simulink model "Robotics_KalmanFilter_example"  (R2022b)
settings: Solver=ode45  StartTime=0.0  StopTime=30  MaxStep=0.01  RelTol=1e-3
libraries: dspmathops x1
settings Model: Creator=score  LastModifiedBy=zhouwenjie
settings OptimizationCC: ReuseModelBlockBuffer=on

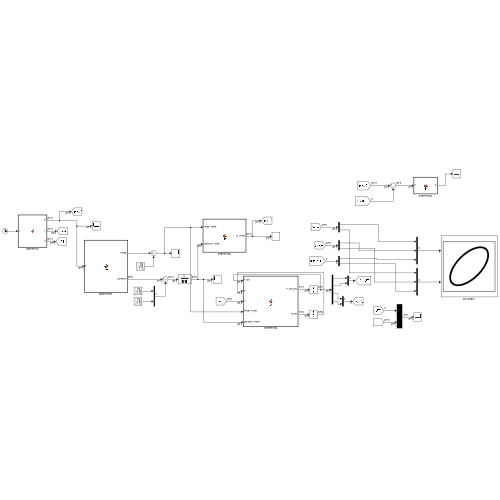
[thumbnail: Simulink's stored preview of the top-level diagram]
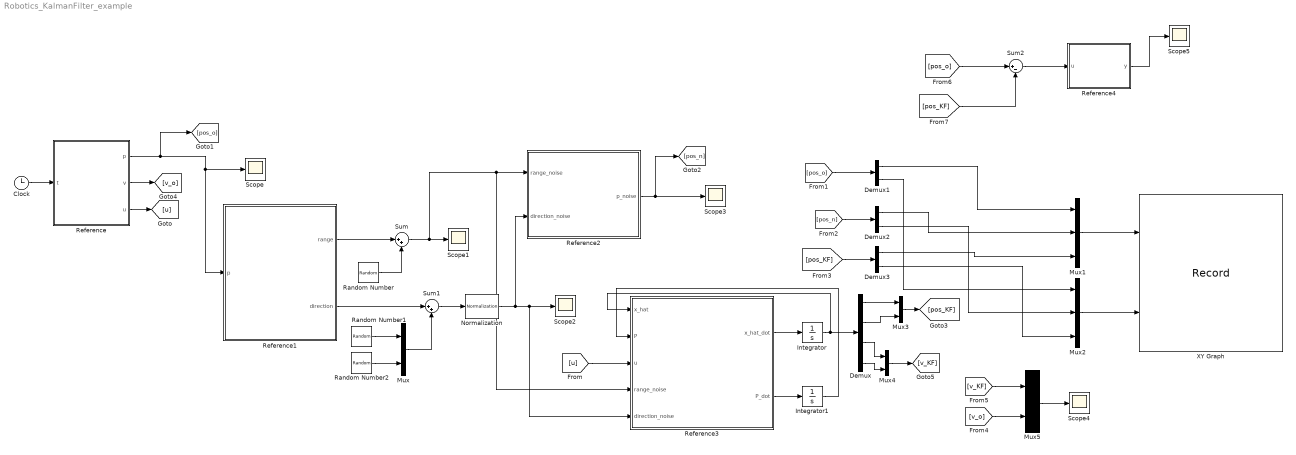
== system Robotics_KalmanFilter_example ==
  Clock : Clock
  Demux : Demux
  Demux1 : Demux  Outputs=2
  Demux2 : Demux  Outputs=2
  Demux3 : Demux  Outputs=2
  Integrator : Integrator  InitialCondition=[-3; -3; 0; 0]
  Integrator1 : Integrator  InitialCondition=100*eye(4)
  Mux{,3..5} (4 alike) : Mux  Inputs=2
  Mux1 : Mux  Inputs=3
  Mux2 : Mux  Inputs=3
  Normalization : dspmathops/Normalization  NormType=2-norm  Bias=1e-10  NormOver=Each column  Dimension=1  roundingMode=Floor  overflowMode=off  accumDataTypeStr=Inherit: Same as product output  accumLastDataTypeStr=Inherit: Same as product output  outputDataTypeStr=Inherit: Same as product output  outputMin=[]  outputMax=[]  outputLastDataTypeStr=Inherit: Same as product output
  Random Number : RandomNumber  Variance=0.01  Seed=randi(1000)  SampleTime=0.01
  Random Number1 : RandomNumber  Variance=0.01  Seed=randi(2000)  SampleTime=0.01
  Random Number2 : RandomNumber  Variance=0.01  Seed=randi(10000)  SampleTime=0.01
  Reference : MATLAB Function  TreatAsAtomicUnit=on
  Reference1 : MATLAB Function  TreatAsAtomicUnit=on
  Reference2 : MATLAB Function  TreatAsAtomicUnit=on
  Reference3 : MATLAB Function  TreatAsAtomicUnit=on
  Reference4 : MATLAB Function  TreatAsAtomicUnit=on
  Scope{,1..5} (6 alike) : Scope
  Sum : Sum  Inputs=|++
  Sum1 : Sum  Inputs=|++
  Sum2 : Sum  Inputs=|+-
  XY Graph : Record  FileSettingsInternal="{\"entries\":[{\"content\":{\"excelSettings\":{\"content\":{},\"type\":\"Streamout.ExcelSettings\"}},\"type\":\"Streamout.FileSettingStorage\",\"uuid\":\"99ddf482-bfd5-4986-8ef2-d08f1135ea4a\"}],\"packageUris\":[\"http://schema.mathworks.com/mf0/streamout_blocks/R2020a\"],\"version\":\"1.0\"}"  Layout=[1 1]  SignalsInternal="{\"entries\":[{\"content\":{\"signals\":[{\"content\":{\"blockPath\":[\"Robotics_KalmanFilter_example/XY Graph\"],\"channel\":[],\"dimensions\":[3],\"domain\":\"Robotics_KalmanFilter_example/XY Graph\",\"hasChildren\":true,\"lineColor\":\"#77ac30\",\"plots\":[],\"port\":1,\"sid\":[\"\"],\"signalID\":486,\"signalName\":\"Mux1\"},\"type\":\"RecordBlkView.Signal\",\"uuid\":\"85c66cea-82c2-4576-a2a4-b02d7115ceed\"},{\"content\":{\"blockPath\":[\"Robotics_KalmanFilter_example/XY Graph\"],\"channel\":[1],\"dimensions\":[3],\"domain\":\"Robotics_KalmanFilter_example/XY Graph\",\"lineColor\":\"#4dbeee\",\"parentID\":486,\"plots\":[1],\"port\":1,\"sid\":[\"\"],\"signalID\":487,\"signalName\":\"Mux1\"},\"type\":\"RecordBlkView.Signal\",\"uuid\":\"cc40eaf1-a560-40e5-9d45-80ed3782b7a2\"},{\"content\":{\"blockPath\":[\"Robotics_KalmanFilter_example/XY Graph\"],\"channel\":[],\"dimensions\":[3],\"domain\":\"Robotics_KalmanFilter_example/XY Graph\",\"hasChildren\":true,\"lineColor\":\"#a2142f\",\"plots\":[],\"port\":2,\"sid\":[\"\"],\"signalID\":491,\"signalName\":\"Mux2\"},\"type\":\"RecordBlkView.Signal\",\"uuid\":\"08abc5d3-c380-4d97-8386-a1200ecf61fc\"},{\"content\":{\"blockPath\":[\"Robotics_KalmanFilter_example/XY Graph\"],\"channel\":[1],\"dimensions\":[3],\"domain\":\"Robotics_KalmanFilter_example/XY Graph\",\"lineColor\":\"#139fff\",\"parentID\":491,\"plots\":[1],\"port\":2,\"sid\":[\"\"],\"signalID\":492,\"signalName\":\"Mux2\"},\"type\":\"RecordBlkView.Signal\",\"uuid\":\"281db55c-b3c3-4430-b4b5-2a782cee91c7\"},{\"content\":{\"blockPath\":[\"Robotics_KalmanFilter_example/XY Graph\"],\"channel\":[2],\"dimensions\":[3],\"domain\":\"Robotics_KalmanFilter_example/XY Graph\",\"lineColor\":\"#ff6929\",\"parentID\":486,\"plots\":[1],\"port\":1,\"sid\":[\"\"],\"signalID\":496,\"signalName\":\"Mux1\"},\"type\":\"RecordBlkView.Signal\",\"uuid\":\"7a39d2fa-2334-4a71-8704-de6660aef924\"},{\"content\":{\"blockPath\":[\"Robotics_KalmanFilter_example/XY Graph\"],\"channel\":[3],\"dimensions\":[3],\"domain\":\"Robotics_KalmanFilter_example/XY Graph\",\"lineColor\":\"#b746ff\",\"parentID\":486,\"plots\":[1],\"port\":1,\"sid\":[\"\"],\"signalID\":497,\"signalName\":\"Mux1\"},\"type\":\"RecordBlkView.Signal\",\"uuid\":\"9c037c13-9f68-4801-a7b2-66cb5fafd5da\"},{\"content\":{\"blockPath\":[\"Robotics_KalmanFilter_example/XY Graph\"],\"channel\":[2],\"dimensions\":[3],\"domain\":\"Robotics_KalmanFilter_example/XY Graph\",\"lineColor\":\"#64d413\",\"parentID\":491,\"plots\":[1],\"port\":2,\"sid\":[\"\"],\"signalID\":498,\"signalName\":\"Mux2\"},\"type\":\"RecordBlkView.Signal\",\"uuid\":\"d5859256-777d-4e96-97fc-4e17bee01a9a\"},{\"content\":{\"blockPath\":[\"Robotics_KalmanFilter_example/XY Graph\"],\"channel\":[3],\"dimensions\":[3],\"domain\":\"Robotics_KalmanFilter_example/XY Graph\",\"lineColor\":\"#ff13a6\",\"parentID\":491,\"plots\":[1],\"port\":2,\"sid\":[\"\"],\"signalID\":499,\"signalName\":\"Mux2\"},\"type\":\"RecordBlkView.Signal\",\"uuid\":\"d73878a8-5330-4d11-8cb2-697f64e39e63\"}]},\"type\":\"RecordBlkView.InputSignals\",\"uuid\":\"f320aaa5-5c90-4b2a-a994-0aa79a653834\"}],\"packageUris\":[\"http://schema.mathworks.com/mf0/streamout_blocks/R2020a\"],\"version\":\"1.0\"}"  VisualizationBindings="{\"xyplotplugin\":{\"info\":[{\"series\":[{\"bindingParametersList\":[{\"parameter\":\"X-Axis\",\"signalID\":496,\"signalName\":\"Mux1(2)\"},{\"parameter\":\"Y-Axis\",\"signalID\":498,\"signalName\":\"Mux2(2)\"}],\"seriesID\":37893},{\"bindingParametersList\":[{\"parameter\":\"X-Axis\",\"signalID\":487,\"signalName\":\"Mux1(1)\"},{\"parameter\":\"Y-Axis\",\"signalID\":492,\"signalName\":\"Mux2(1)\"}],\"seriesID\":24155},{\"bindingParametersList\":[{\"parameter\":\"X-Axis\",\"signalID\":497,\"signalName\":\"Mux1(3)\"},{\"parameter\":\"Y-Axis\",\"signalID\":499,\"signalName\":\"Mux2(3)\"}],\"seriesID\":670}],\"subplotID\":1}]}}"  CompatibilityTag=XY
  wires:
  Clock/1 -> Reference/1(t)
  Reference/1(p) -> [pos_o], Reference1/1(p), Scope/1
  Reference1/1(range) -> Sum/1
  Random Number/1 -> Sum/2
  Reference1/2(direction) -> Sum1/1
  Random Number1/1 -> Mux/1
  Random Number2/1 -> Mux/2
  Mux/1 -> Sum1/2
  Sum1/1 -> Normalization/1
  Sum/1 -> Reference2/1(range_noise), Reference3/4(range_noise), Scope1/1
  Normalization/1 -> Reference2/2(direction_noise), Reference3/5(direction_noise), Scope2/1
  Reference2/1(p_noise) -> [pos_n], Scope3/1
  Reference3/1(x_hat_dot) -> Integrator/1
  Reference3/2(P_dot) -> Integrator1/1
  Integrator1/1 -> Reference3/2(P)
  Integrator/1 -> Reference3/1(x_hat), Demux/1
  Reference/3(u) -> [u]
  [u] -> Reference3/3(u)
  Mux1/1 -> XY Graph/1
  Mux2/1 -> XY Graph/2
  Demux/1 -> Mux3/1
  Demux/2 -> Mux3/2
  Mux3/1 -> [pos_KF]
  [pos_o] -> Demux1/1
  [pos_n] -> Demux2/1
  [pos_KF] -> Demux3/1
  Demux1/1 -> Mux1/1
  Demux2/1 -> Mux1/2
  Demux3/1 -> Mux1/3
  Demux1/2 -> Mux2/1
  Demux2/2 -> Mux2/2
  Demux3/2 -> Mux2/3
  Reference/2(v) -> [v_o]
  Demux/3 -> Mux4/1
  Mux4/1 -> [v_KF]
  Demux/4 -> Mux4/2
  [v_KF] -> Mux5/1
  [v_o] -> Mux5/2
  Mux5/1 -> Scope4/1
  [pos_o] -> Sum2/1
  [pos_KF] -> Sum2/2
  Sum2/1 -> Reference4/1(u)
  Reference4/1(y) -> Scope5/1

== matlab function Robotics_KalmanFilter_example/Reference1 ==
  data: p input; range output; direction output
function [range, direction] = fcn(p)

range = norm(p);
direction = p/range;

== matlab function Robotics_KalmanFilter_example/Reference ==
  data: t input; p output; v output; u output
function [p, v, u] = fcn(t)

a = 1/2;
b = 1;
alpha = 1;
beta = -1/3;

p = [a*cos(alpha*t);
     b*sin(beta*t)];

v = [-a*alpha*sin(alpha*t);
     b*beta*cos(beta*t)];

u = [-a*alpha^2*cos(alpha*t);
     -b*beta^2*sin(beta*t)];

== matlab function Robotics_KalmanFilter_example/Reference2 ==
  data: range_noise input; p_noise output; direction_noise input
function p_noise = fcn(range_noise, direction_noise)

p_noise = range_noise*direction_noise;

== matlab function Robotics_KalmanFilter_example/Reference3 ==
  data: x_hat input; P input; u input; range_noise input; x_hat_dot output; direction_noise input; P_dot output
function [x_hat_dot, P_dot] = fcn(x_hat, P, u, range_noise, direction_noise)

A = [zeros(2), eye(2);
     zeros(2), zeros(2)];

C = [eye(2), zeros(2)];

Q = 1e-7*eye(4);
R = 10*eye(2);

y = range_noise*direction_noise;

K = P*C'/R;

x_hat_dot = A*x_hat + [zeros(2,1); u] + K*(y - C*x_hat);

P_dot = A*P + P*A' + Q - K*R*K';

== matlab function Robotics_KalmanFilter_example/Reference4 ==
  data: u input; y output
function y = fcn(u)

y = norm(u);
